simulink model "FirmwareArchitecture"  (R2024a)
settings: Solver=FixedStepDiscrete  StartTime=0.0  StopTime=10.0  RelTol=1e-3
model workspace (MAT data in the model file):
  AuralSystemInterface = Simulink.ServiceBus
  AuralSystemInterface.Elements_internal(1) = Simulink.FunctionElement
  AuralSystemInterface.Elements_internal(1).Prototype = 'vAuralSystemInit()'
  AuralSystemInterface.Elements_internal(1).Name = 'vAuralSystemInit'
  AuralSystemInterface.Elements_internal(1).Asynchronous = 0
  AuralSystemInterface.Elements_internal(2) = Simulink.FunctionElement
  AuralSystemInterface.Elements_internal(2).Prototype = 'vAuralSystemPlayWarningLevelChime()'
  AuralSystemInterface.Elements_internal(2).Name = 'vAuralSystemPlayWarningLevelChime'
  AuralSystemInterface.Elements_internal(2).Asynchronous = 0
  AuralSystemInterface.Elements_internal(3) = Simulink.FunctionElement
  AuralSystemInterface.Elements_internal(3).Prototype = 'vAuralSystemPlayFaultLevelChime()'
  AuralSystemInterface.Elements_internal(3).Name = 'vAuralSystemPlayFaultLevelChime'
  AuralSystemInterface.Elements_internal(3).Asynchronous = 0
  CollisionSensorInterface = Simulink.ServiceBus
  CollisionSensorInterface.Elements_internal(1) = Simulink.FunctionElement
  CollisionSensorInterface.Elements_internal(1).Prototype = 'vCollisionSensorInit(pCollisionCallBack)'
  CollisionSensorInterface.Elements_internal(1).Name = 'vCollisionSensorInit'
  CollisionSensorInterface.Elements_internal(1).Asynchronous = 0
  CollisionSensorInterface.Elements_internal(1).Arguments = Simulink.BusElement
  CollisionSensorInterface.Elements_internal(1).Arguments.DimensionsMode = 'Fixed'
  CollisionSensorInterface.Elements_internal(1).Arguments.SamplingMode = 'Sample based'
  CollisionSensorInterface.Elements_internal(1).Arguments.SampleTime = -1
  CollisionSensorInterface.Elements_internal(1).Arguments.Description = 'Pointer to Callback function'
  CollisionSensorInterface.Elements_internal(1).Arguments.Name = 'pCollisionCallBack'
  CollisionSensorInterface.Elements_internal(1).Arguments.DataType_internal = 'void (*)'
  CollisionSensorInterface.Elements_internal(1).Arguments.Complexity = 'real'
  CollisionSensorInterface.Elements_internal(1).Arguments.Dimensions = 1
  CollisionSensorInterface.Elements_internal(2) = Simulink.FunctionElement
  CollisionSensorInterface.Elements_internal(2).Prototype = 'vCollisionSensorDetectionHandler()'
  CollisionSensorInterface.Elements_internal(2).Name = 'vCollisionSensorDetectionHandler'
  CollisionSensorInterface.Elements_internal(2).Asynchronous = 0
  EncoderSystemInterface = Simulink.ServiceBus
  EncoderSystemInterface.Elements_internal(1) = Simulink.FunctionElement
  EncoderSystemInterface.Elements_internal(1).Prototype = 'vEncoderSystemInit(pLeftMotorCount,pRightMotorCount)'
  EncoderSystemInterface.Elements_internal(1).Name = 'vEncoderSystemInit'
  EncoderSystemInterface.Elements_internal(1).Asynchronous = 0
  EncoderSystemInterface.Elements_internal(1).Arguments(1) = Simulink.BusElement
  EncoderSystemInterface.Elements_internal(1).Arguments(1).DimensionsMode = 'Fixed'
  EncoderSystemInterface.Elements_internal(1).Arguments(1).SamplingMode = 'Sample based'
  EncoderSystemInterface.Elements_internal(1).Arguments(1).SampleTime = -1
  EncoderSystemInterface.Elements_internal(1).Arguments(1).Name = 'pLeftMotorCount'
  EncoderSystemInterface.Elements_internal(1).Arguments(1).DataType_internal = 'unsigned int*'
  EncoderSystemInterface.Elements_internal(1).Arguments(1).Complexity = 'real'
  EncoderSystemInterface.Elements_internal(1).Arguments(1).Dimensions = 1
  EncoderSystemInterface.Elements_internal(1).Arguments(2) = Simulink.BusElement
  EncoderSystemInterface.Elements_internal(1).Arguments(2).DimensionsMode = 'Fixed'
  EncoderSystemInterface.Elements_internal(1).Arguments(2).SamplingMode = 'Sample based'
  EncoderSystemInterface.Elements_internal(1).Arguments(2).SampleTime = -1
  EncoderSystemInterface.Elements_internal(1).Arguments(2).Name = 'pRightMotorCount'
  EncoderSystemInterface.Elements_internal(1).Arguments(2).DataType_internal = 'unsigned int*'
  EncoderSystemInterface.Elements_internal(1).Arguments(2).Complexity = 'real'
  EncoderSystemInterface.Elements_internal(1).Arguments(2).Dimensions = 1
  EncoderSystemInterface.Elements_internal(2) = Simulink.FunctionElement
  EncoderSystemInterface.Elements_internal(2).Prototype = 'vEncoderSystemExecuteMeasurement()'
  EncoderSystemInterface.Elements_internal(2).Name = 'vEncoderSystemExecuteMeasurement'
  EncoderSystemInterface.Elements_internal(2).Asynchronous = 0
  InfraredDistanceSystemInterface = Simulink.ServiceBus
  InfraredDistanceSystemInterface.Elements_internal(1) = Simulink.FunctionElement
  InfraredDistanceSystemInterface.Elements_internal(1).Prototype = 'vInfraredDistanceSystemInit(pDistanceMeasurement)'
  InfraredDistanceSystemInterface.Elements_internal(1).Name = 'vInfraredDistanceSystemInit'
  InfraredDistanceSystemInterface.Elements_internal(1).Asynchronous = 0
  InfraredDistanceSystemInterface.Elements_internal(1).Arguments = Simulink.BusElement
  InfraredDistanceSystemInterface.Elements_internal(1).Arguments.DimensionsMode = 'Fixed'
  InfraredDistanceSystemInterface.Elements_internal(1).Arguments.SamplingMode = 'Sample based'
  InfraredDistanceSystemInterface.Elements_internal(1).Arguments.SampleTime = -1
  InfraredDistanceSystemInterface.Elements_internal(1).Arguments.Name = 'pDistanceMeasurement'
  InfraredDistanceSystemInterface.Elements_internal(1).Arguments.DataType_internal = 'float*'
  InfraredDistanceSystemInterface.Elements_internal(1).Arguments.Complexity = 'real'
  InfraredDistanceSystemInterface.Elements_internal(1).Arguments.Dimensions = 1
  InfraredDistanceSystemInterface.Elements_internal(2) = Simulink.FunctionElement
  InfraredDistanceSystemInterface.Elements_internal(2).Prototype = 'vInfraredDistanceSystemExcecuteMeasurement()'
  InfraredDistanceSystemInterface.Elements_internal(2).Name = 'vInfraredDistanceSystemExcecuteMeasurement'
  InfraredDistanceSystemInterface.Elements_internal(2).Asynchronous = 0
  LineSensorSystemInterface = Simulink.ServiceBus
  LineSensorSystemInterface.Elements_internal = Simulink.FunctionElement
  LineSensorSystemInterface.Elements_internal.Prototype = 'LineSensorSystemInit(pLineSensorsReadings)'
  LineSensorSystemInterface.Elements_internal.Name = 'LineSensorSystemInit'
  LineSensorSystemInterface.Elements_internal.Asynchronous = 0
  LineSensorSystemInterface.Elements_internal.Arguments = Simulink.BusElement
  LineSensorSystemInterface.Elements_internal.Arguments.DimensionsMode = 'Fixed'
  LineSensorSystemInterface.Elements_internal.Arguments.SamplingMode = 'Sample based'
  LineSensorSystemInterface.Elements_internal.Arguments.SampleTime = -1
  LineSensorSystemInterface.Elements_internal.Arguments.Name = 'pLineSensorsReadings'
  LineSensorSystemInterface.Elements_internal.Arguments.DataType_internal = 'long unsigned int* [5]'
  LineSensorSystemInterface.Elements_internal.Arguments.Complexity = 'real'
  LineSensorSystemInterface.Elements_internal.Arguments.Dimensions = 5
  TelemetrySystemInterface = Simulink.ServiceBus
  TelemetrySystemInterface.Elements_internal(1) = Simulink.FunctionElement
  TelemetrySystemInterface.Elements_internal(1).Prototype = 'vTelemetrySystemInit()'
  TelemetrySystemInterface.Elements_internal(1).Name = 'vTelemetrySystemInit'
  TelemetrySystemInterface.Elements_internal(1).Asynchronous = 0
  TelemetrySystemInterface.Elements_internal(2) = Simulink.FunctionElement
  TelemetrySystemInterface.Elements_internal(2).Prototype = 'vTelemetrySystemSchedullingHandler(pTIM)'
  TelemetrySystemInterface.Elements_internal(2).Name = 'vTelemetrySystemSchedullingHandler'
  TelemetrySystemInterface.Elements_internal(2).Asynchronous = 1
  TelemetrySystemInterface.Elements_internal(2).Arguments = Simulink.BusElement
  TelemetrySystemInterface.Elements_internal(2).Arguments.DimensionsMode = 'Fixed'
  TelemetrySystemInterface.Elements_internal(2).Arguments.SamplingMode = 'Sample based'
  TelemetrySystemInterface.Elements_internal(2).Arguments.SampleTime = -1
  TelemetrySystemInterface.Elements_internal(2).Arguments.Name = 'pTIM'
  TelemetrySystemInterface.Elements_internal(2).Arguments.DataType_internal = 'TIM_HandleTypeDef*'
  TelemetrySystemInterface.Elements_internal(2).Arguments.Complexity = 'real'
  TelemetrySystemInterface.Elements_internal(2).Arguments.Dimensions = 1
  TelemetrySystemInterface.Elements_internal(3) = Simulink.FunctionElement
  TelemetrySystemInterface.Elements_internal(3).Prototype = 'vTelemetrySystemExternalEventHandler(uiGpioPin)'
  TelemetrySystemInterface.Elements_internal(3).Name = 'vTelemetrySystemExternalEventHandler'
  TelemetrySystemInterface.Elements_internal(3).Asynchronous = 1
  TelemetrySystemInterface.Elements_internal(3).Arguments = Simulink.BusElement
  TelemetrySystemInterface.Elements_internal(3).Arguments.DimensionsMode = 'Fixed'
  TelemetrySystemInterface.Elements_internal(3).Arguments.SamplingMode = 'Sample based'
  TelemetrySystemInterface.Elements_internal(3).Arguments.SampleTime = -1
  TelemetrySystemInterface.Elements_internal(3).Arguments.Name = 'uiGpioPin'
  TelemetrySystemInterface.Elements_internal(3).Arguments.DataType_internal = 'uint16'
  TelemetrySystemInterface.Elements_internal(3).Arguments.Complexity = 'real'
  TelemetrySystemInterface.Elements_internal(3).Arguments.Dimensions = 1
  UltrassonicDistanceSystemInterface = Simulink.ServiceBus
  UltrassonicDistanceSystemInterface.Elements_internal(1) = Simulink.FunctionElement
  UltrassonicDistanceSystemInterface.Elements_internal(1).Prototype = 'vUltrassonicDistanceSystemInit(pDistanceMeasurement)'
  UltrassonicDistanceSystemInterface.Elements_internal(1).Name = 'vUltrassonicDistanceSystemInit'
  UltrassonicDistanceSystemInterface.Elements_internal(1).Asynchronous = 0
  UltrassonicDistanceSystemInterface.Elements_internal(1).Arguments = Simulink.BusElement
  UltrassonicDistanceSystemInterface.Elements_internal(1).Arguments.DimensionsMode = 'Fixed'
  UltrassonicDistanceSystemInterface.Elements_internal(1).Arguments.SamplingMode = 'Sample based'
  UltrassonicDistanceSystemInterface.Elements_internal(1).Arguments.SampleTime = -1
  UltrassonicDistanceSystemInterface.Elements_internal(1).Arguments.Name = 'pDistanceMeasurement'
  UltrassonicDistanceSystemInterface.Elements_internal(1).Arguments.DataType_internal = 'float*'
  UltrassonicDistanceSystemInterface.Elements_internal(1).Arguments.Complexity = 'real'
  UltrassonicDistanceSystemInterface.Elements_internal(1).Arguments.Dimensions = 1
  UltrassonicDistanceSystemInterface.Elements_internal(2) = Simulink.FunctionElement
  UltrassonicDistanceSystemInterface.Elements_internal(2).Prototype = 'vUltrassonicDistanceSystemExecuteMeasurement()'
  UltrassonicDistanceSystemInterface.Elements_internal(2).Name = 'vUltrassonicDistanceSystemExecuteMeasurement'
  UltrassonicDistanceSystemInterface.Elements_internal(2).Asynchronous = 0
  UltrassonicDistanceSystemInterface.Elements_internal(3) = Simulink.FunctionElement
  UltrassonicDistanceSystemInterface.Elements_internal(3).Prototype = 'vUltrassonicDistanceSystemPulseHandler()'
  UltrassonicDistanceSystemInterface.Elements_internal(3).Name = 'vUltrassonicDistanceSystemPulseHandler'
  UltrassonicDistanceSystemInterface.Elements_internal(3).Asynchronous = 1
settings Model: Creator=pedro  LastModifiedBy=pedro

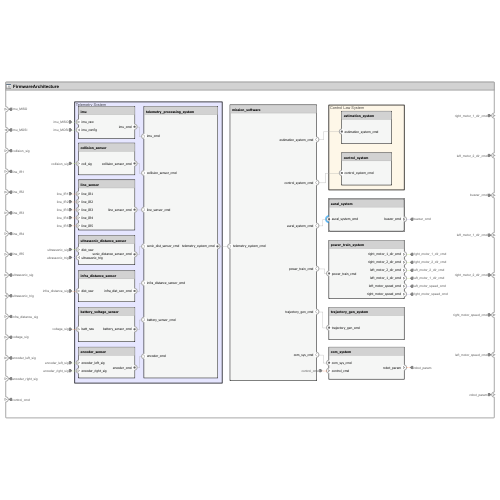
[thumbnail: Simulink's stored preview of the top-level diagram]
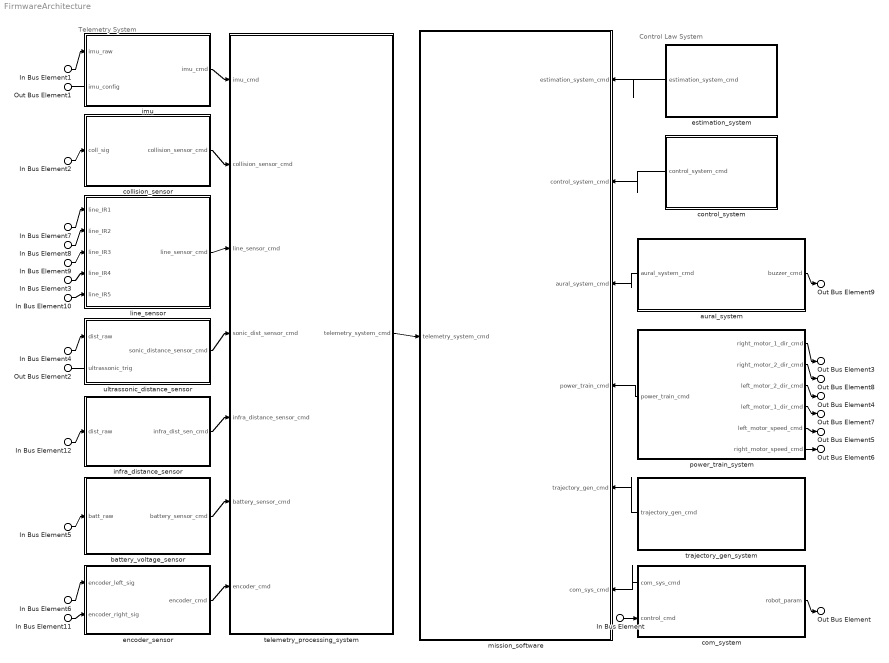
== system FirmwareArchitecture ==
  note: Control Law System
  note: Telemetry System
  In Bus Element1 : Inport  PortName=imu_MISO
  In Bus Element2 : Inport  Port=2  PortName=collision_sig
  In Bus Element7 : Inport  Port=3  PortName=line_IR1
  In Bus Element8 : Inport  Port=4  PortName=line_IR2
  In Bus Element9 : Inport  Port=5  PortName=line_IR3
  In Bus Element3 : Inport  Port=6  PortName=line_IR4
  In Bus Element10 : Inport  Port=7  PortName=line_IR5
  In Bus Element4 : Inport  Port=8  PortName=ultrassonic_sig
  In Bus Element5 : Inport  Port=9  PortName=voltage_sig
  In Bus Element12 : Inport  Port=10  PortName=infra_distance_sig
  In Bus Element6 : Inport  Port=11  PortName=encoder_left_sig
  In Bus Element11 : Inport  Port=12  PortName=encoder_right_sig
  In Bus Element : Inport  Port=13  PortName=control_cmd
  aural_system : Subsystem
      settings: PortSchema="{\"entries\":[{\"content\":{\"headerSize\":26,\"margin\":15,\"minimumSpacing\":25,\"sides\":[{\"content\":{\"connectorIds\":[\"Out2\"]},\"type\":\"ConnectorPlacement.EquallySpacedRectSide\",\"uuid\":\"4d6c5e10-6186-41fb-b2bf-ba98d7aba04e\"},{\"content\":{\"connectorIds\":[\"Out1\"],\"side\":\"RIGHT\"},\"type\":\"ConnectorPlacement.EquallySpacedRectSide\",\"uuid\":\"376cbcb5-ae00-4ee4-b51a-d7e41488d4d0\"},{\"content\":{\"side\":\"TOP\"},\"type\":\"ConnectorPlacement.EquallySpacedRectSide\",\"uuid\":\"7d78b6f2-ded8-4819-b676-701e54dd8720\"}]},\"type\":\"ConnectorPlacement.EquallySpacedConnector\",\"uuid\":\"61036d85-7ed2-4698-95df-f6a26735d595\"}],\"packageUris\":[\"http://schema.mathworks.com/mf0/Connector/R2020b\"],\"version\":\"1.0\"}"
  battery_voltage_sensor : Subsystem
      settings: PortSchema="{\"entries\":[{\"content\":{\"headerSize\":26,\"margin\":15,\"minimumSpacing\":25,\"sides\":[{\"content\":{\"connectorIds\":[\"In1\"]},\"type\":\"ConnectorPlacement.EquallySpacedRectSide\",\"uuid\":\"4d6c5e10-6186-41fb-b2bf-ba98d7aba04e\"},{\"content\":{\"connectorIds\":[\"Out1\"],\"side\":\"RIGHT\"},\"type\":\"ConnectorPlacement.EquallySpacedRectSide\",\"uuid\":\"376cbcb5-ae00-4ee4-b51a-d7e41488d4d0\"},{\"content\":{\"side\":\"TOP\"},\"type\":\"ConnectorPlacement.EquallySpacedRectSide\",\"uuid\":\"7d78b6f2-ded8-4819-b676-701e54dd8720\"}]},\"type\":\"ConnectorPlacement.EquallySpacedConnector\",\"uuid\":\"61036d85-7ed2-4698-95df-f6a26735d595\"}],\"packageUris\":[\"http://schema.mathworks.com/mf0/Connector/R2020b\"],\"version\":\"1.0\"}"
  collision_sensor : Subsystem
      settings: PortSchema="{\"entries\":[{\"content\":{\"headerSize\":26,\"margin\":15,\"minimumSpacing\":25,\"sides\":[{\"content\":{\"connectorIds\":[\"In1\"]},\"type\":\"ConnectorPlacement.EquallySpacedRectSide\",\"uuid\":\"4d6c5e10-6186-41fb-b2bf-ba98d7aba04e\"},{\"content\":{\"connectorIds\":[\"Out1\"],\"side\":\"RIGHT\"},\"type\":\"ConnectorPlacement.EquallySpacedRectSide\",\"uuid\":\"376cbcb5-ae00-4ee4-b51a-d7e41488d4d0\"},{\"content\":{\"side\":\"TOP\"},\"type\":\"ConnectorPlacement.EquallySpacedRectSide\",\"uuid\":\"7d78b6f2-ded8-4819-b676-701e54dd8720\"}]},\"type\":\"ConnectorPlacement.EquallySpacedConnector\",\"uuid\":\"61036d85-7ed2-4698-95df-f6a26735d595\"}],\"packageUris\":[\"http://schema.mathworks.com/mf0/Connector/R2020b\"],\"version\":\"1.0\"}"
  com_system : Subsystem
      settings: PortSchema="{\"entries\":[{\"content\":{\"headerSize\":26,\"margin\":15,\"minimumSpacing\":25,\"sides\":[{\"content\":{\"connectorIds\":[\"Out2\",\"In1\"]},\"type\":\"ConnectorPlacement.EquallySpacedRectSide\",\"uuid\":\"4d6c5e10-6186-41fb-b2bf-ba98d7aba04e\"},{\"content\":{\"connectorIds\":[\"Out1\"],\"side\":\"RIGHT\"},\"type\":\"ConnectorPlacement.EquallySpacedRectSide\",\"uuid\":\"376cbcb5-ae00-4ee4-b51a-d7e41488d4d0\"},{\"content\":{\"side\":\"TOP\"},\"type\":\"ConnectorPlacement.EquallySpacedRectSide\",\"uuid\":\"7d78b6f2-ded8-4819-b676-701e54dd8720\"}]},\"type\":\"ConnectorPlacement.EquallySpacedConnector\",\"uuid\":\"61036d85-7ed2-4698-95df-f6a26735d595\"}],\"packageUris\":[\"http://schema.mathworks.com/mf0/Connector/R2020b\"],\"version\":\"1.0\"}"
  control_system : Subsystem
      settings: PortSchema="{\"entries\":[{\"content\":{\"headerSize\":26,\"margin\":15,\"minimumSpacing\":25,\"sides\":[{\"content\":{\"connectorIds\":[\"Out1\"]},\"type\":\"ConnectorPlacement.EquallySpacedRectSide\",\"uuid\":\"4d6c5e10-6186-41fb-b2bf-ba98d7aba04e\"},{\"content\":{\"side\":\"RIGHT\"},\"type\":\"ConnectorPlacement.EquallySpacedRectSide\",\"uuid\":\"376cbcb5-ae00-4ee4-b51a-d7e41488d4d0\"},{\"content\":{\"side\":\"TOP\"},\"type\":\"ConnectorPlacement.EquallySpacedRectSide\",\"uuid\":\"7d78b6f2-ded8-4819-b676-701e54dd8720\"}]},\"type\":\"ConnectorPlacement.EquallySpacedConnector\",\"uuid\":\"61036d85-7ed2-4698-95df-f6a26735d595\"}],\"packageUris\":[\"http://schema.mathworks.com/mf0/Connector/R2020b\"],\"version\":\"1.0\"}"
  encoder_sensor : Subsystem
      settings: PortSchema="{\"entries\":[{\"content\":{\"headerSize\":26,\"margin\":15,\"minimumSpacing\":25,\"sides\":[{\"content\":{\"connectorIds\":[\"In1\",\"In2\"]},\"type\":\"ConnectorPlacement.EquallySpacedRectSide\",\"uuid\":\"4d6c5e10-6186-41fb-b2bf-ba98d7aba04e\"},{\"content\":{\"connectorIds\":[\"Out1\"],\"side\":\"RIGHT\"},\"type\":\"ConnectorPlacement.EquallySpacedRectSide\",\"uuid\":\"376cbcb5-ae00-4ee4-b51a-d7e41488d4d0\"},{\"content\":{\"side\":\"TOP\"},\"type\":\"ConnectorPlacement.EquallySpacedRectSide\",\"uuid\":\"7d78b6f2-ded8-4819-b676-701e54dd8720\"}]},\"type\":\"ConnectorPlacement.EquallySpacedConnector\",\"uuid\":\"61036d85-7ed2-4698-95df-f6a26735d595\"}],\"packageUris\":[\"http://schema.mathworks.com/mf0/Connector/R2020b\"],\"version\":\"1.0\"}"
  estimation_system : Subsystem
      settings: PortSchema="{\"entries\":[{\"content\":{\"headerSize\":26,\"margin\":15,\"minimumSpacing\":25,\"sides\":[{\"content\":{\"connectorIds\":[\"Out1\"]},\"type\":\"ConnectorPlacement.EquallySpacedRectSide\",\"uuid\":\"4d6c5e10-6186-41fb-b2bf-ba98d7aba04e\"},{\"content\":{\"side\":\"RIGHT\"},\"type\":\"ConnectorPlacement.EquallySpacedRectSide\",\"uuid\":\"376cbcb5-ae00-4ee4-b51a-d7e41488d4d0\"},{\"content\":{\"side\":\"TOP\"},\"type\":\"ConnectorPlacement.EquallySpacedRectSide\",\"uuid\":\"7d78b6f2-ded8-4819-b676-701e54dd8720\"}]},\"type\":\"ConnectorPlacement.EquallySpacedConnector\",\"uuid\":\"61036d85-7ed2-4698-95df-f6a26735d595\"}],\"packageUris\":[\"http://schema.mathworks.com/mf0/Connector/R2020b\"],\"version\":\"1.0\"}"
  imu : Subsystem
      settings: PortSchema="{\"entries\":[{\"content\":{\"headerSize\":26,\"margin\":15,\"minimumSpacing\":25,\"sides\":[{\"content\":{\"connectorIds\":[\"In1\",\"Out2\"]},\"type\":\"ConnectorPlacement.EquallySpacedRectSide\",\"uuid\":\"4d6c5e10-6186-41fb-b2bf-ba98d7aba04e\"},{\"content\":{\"connectorIds\":[\"Out1\"],\"side\":\"RIGHT\"},\"type\":\"ConnectorPlacement.EquallySpacedRectSide\",\"uuid\":\"376cbcb5-ae00-4ee4-b51a-d7e41488d4d0\"},{\"content\":{\"side\":\"TOP\"},\"type\":\"ConnectorPlacement.EquallySpacedRectSide\",\"uuid\":\"7d78b6f2-ded8-4819-b676-701e54dd8720\"}]},\"type\":\"ConnectorPlacement.EquallySpacedConnector\",\"uuid\":\"61036d85-7ed2-4698-95df-f6a26735d595\"}],\"packageUris\":[\"http://schema.mathworks.com/mf0/Connector/R2020b\"],\"version\":\"1.0\"}"
  infra_distance_sensor : Subsystem
      settings: PortSchema="{\"entries\":[{\"content\":{\"headerSize\":26,\"margin\":15,\"minimumSpacing\":25,\"sides\":[{\"content\":{\"connectorIds\":[\"In1\"]},\"type\":\"ConnectorPlacement.EquallySpacedRectSide\",\"uuid\":\"4d6c5e10-6186-41fb-b2bf-ba98d7aba04e\"},{\"content\":{\"connectorIds\":[\"Out1\"],\"side\":\"RIGHT\"},\"type\":\"ConnectorPlacement.EquallySpacedRectSide\",\"uuid\":\"376cbcb5-ae00-4ee4-b51a-d7e41488d4d0\"},{\"content\":{\"side\":\"TOP\"},\"type\":\"ConnectorPlacement.EquallySpacedRectSide\",\"uuid\":\"7d78b6f2-ded8-4819-b676-701e54dd8720\"}]},\"type\":\"ConnectorPlacement.EquallySpacedConnector\",\"uuid\":\"61036d85-7ed2-4698-95df-f6a26735d595\"}],\"packageUris\":[\"http://schema.mathworks.com/mf0/Connector/R2020b\"],\"version\":\"1.0\"}"
  line_sensor : Subsystem
      settings: PortSchema="{\"entries\":[{\"content\":{\"headerSize\":26,\"margin\":15,\"minimumSpacing\":25,\"sides\":[{\"content\":{\"connectorIds\":[\"In1\",\"In2\",\"In3\",\"In4\",\"In5\"]},\"type\":\"ConnectorPlacement.EquallySpacedRectSide\",\"uuid\":\"4d6c5e10-6186-41fb-b2bf-ba98d7aba04e\"},{\"content\":{\"connectorIds\":[\"Out1\"],\"side\":\"RIGHT\"},\"type\":\"ConnectorPlacement.EquallySpacedRectSide\",\"uuid\":\"376cbcb5-ae00-4ee4-b51a-d7e41488d4d0\"},{\"content\":{\"side\":\"TOP\"},\"type\":\"ConnectorPlacement.EquallySpacedRectSide\",\"uuid\":\"7d78b6f2-ded8-4819-b676-701e54dd8720\"}]},\"type\":\"ConnectorPlacement.EquallySpacedConnector\",\"uuid\":\"61036d85-7ed2-4698-95df-f6a26735d595\"}],\"packageUris\":[\"http://schema.mathworks.com/mf0/Connector/R2020b\"],\"version\":\"1.0\"}"
  mission_software : Subsystem
      settings: PortSchema="{\"entries\":[{\"content\":{\"headerSize\":26,\"margin\":15,\"minimumSpacing\":25,\"sides\":[{\"content\":{\"connectorIds\":[\"In6\"]},\"type\":\"ConnectorPlacement.EquallySpacedRectSide\",\"uuid\":\"4d6c5e10-6186-41fb-b2bf-ba98d7aba04e\"},{\"content\":{\"connectorIds\":[\"In1\",\"In2\",\"In3\",\"In4\",\"In5\",\"In7\"],\"side\":\"RIGHT\"},\"type\":\"ConnectorPlacement.EquallySpacedRectSide\",\"uuid\":\"376cbcb5-ae00-4ee4-b51a-d7e41488d4d0\"},{\"content\":{\"side\":\"TOP\"},\"type\":\"ConnectorPlacement.EquallySpacedRectSide\",\"uuid\":\"7d78b6f2-ded8-4819-b676-701e54dd8720\"}]},\"type\":\"ConnectorPlacement.EquallySpacedConnector\",\"uuid\":\"61036d85-7ed2-4698-95df-f6a26735d595\"}],\"packageUris\":[\"http://schema.mathworks.com/mf0/Connector/R2020b\"],\"version\":\"1.0\"}"
  power_train_system : Subsystem
      settings: PortSchema="{\"entries\":[{\"content\":{\"headerSize\":26,\"margin\":15,\"minimumSpacing\":25,\"sides\":[{\"content\":{\"connectorIds\":[\"Out7\"]},\"type\":\"ConnectorPlacement.EquallySpacedRectSide\",\"uuid\":\"4d6c5e10-6186-41fb-b2bf-ba98d7aba04e\"},{\"content\":{\"connectorIds\":[\"Out1\",\"Out4\",\"Out2\",\"Out3\",\"Out6\",\"Out5\"],\"side\":\"RIGHT\"},\"type\":\"ConnectorPlacement.EquallySpacedRectSide\",\"uuid\":\"376cbcb5-ae00-4ee4-b51a-d7e41488d4d0\"},{\"content\":{\"side\":\"TOP\"},\"type\":\"ConnectorPlacement.EquallySpacedRectSide\",\"uuid\":\"7d78b6f2-ded8-4819-b676-701e54dd8720\"}]},\"type\":\"ConnectorPlacement.EquallySpacedConnector\",\"uuid\":\"61036d85-7ed2-4698-95df-f6a26735d595\"}],\"packageUris\":[\"http://schema.mathworks.com/mf0/Connector/R2020b\"],\"version\":\"1.0\"}"
  telemetry_processing_system : Subsystem
      settings: PortSchema="{\"entries\":[{\"content\":{\"headerSize\":26,\"margin\":15,\"minimumSpacing\":25,\"sides\":[{\"content\":{\"connectorIds\":[\"In1\",\"In3\",\"In2\",\"In4\",\"In5\",\"In6\",\"In7\"]},\"type\":\"ConnectorPlacement.EquallySpacedRectSide\",\"uuid\":\"4d6c5e10-6186-41fb-b2bf-ba98d7aba04e\"},{\"content\":{\"connectorIds\":[\"Out1\"],\"side\":\"RIGHT\"},\"type\":\"ConnectorPlacement.EquallySpacedRectSide\",\"uuid\":\"376cbcb5-ae00-4ee4-b51a-d7e41488d4d0\"},{\"content\":{\"side\":\"TOP\"},\"type\":\"ConnectorPlacement.EquallySpacedRectSide\",\"uuid\":\"7d78b6f2-ded8-4819-b676-701e54dd8720\"}]},\"type\":\"ConnectorPlacement.EquallySpacedConnector\",\"uuid\":\"61036d85-7ed2-4698-95df-f6a26735d595\"}],\"packageUris\":[\"http://schema.mathworks.com/mf0/Connector/R2020b\"],\"version\":\"1.0\"}"
  trajectory_gen_system : Subsystem
      settings: PortSchema="{\"entries\":[{\"content\":{\"headerSize\":26,\"margin\":15,\"minimumSpacing\":25,\"sides\":[{\"content\":{\"connectorIds\":[\"Out1\"]},\"type\":\"ConnectorPlacement.EquallySpacedRectSide\",\"uuid\":\"4d6c5e10-6186-41fb-b2bf-ba98d7aba04e\"},{\"content\":{\"side\":\"RIGHT\"},\"type\":\"ConnectorPlacement.EquallySpacedRectSide\",\"uuid\":\"376cbcb5-ae00-4ee4-b51a-d7e41488d4d0\"},{\"content\":{\"side\":\"TOP\"},\"type\":\"ConnectorPlacement.EquallySpacedRectSide\",\"uuid\":\"7d78b6f2-ded8-4819-b676-701e54dd8720\"}]},\"type\":\"ConnectorPlacement.EquallySpacedConnector\",\"uuid\":\"61036d85-7ed2-4698-95df-f6a26735d595\"}],\"packageUris\":[\"http://schema.mathworks.com/mf0/Connector/R2020b\"],\"version\":\"1.0\"}"
  ultrassonic_distance_sensor : Subsystem
      settings: PortSchema="{\"entries\":[{\"content\":{\"headerSize\":26,\"margin\":15,\"minimumSpacing\":25,\"sides\":[{\"content\":{\"connectorIds\":[\"In1\",\"Out2\"]},\"type\":\"ConnectorPlacement.EquallySpacedRectSide\",\"uuid\":\"4d6c5e10-6186-41fb-b2bf-ba98d7aba04e\"},{\"content\":{\"connectorIds\":[\"Out1\"],\"side\":\"RIGHT\"},\"type\":\"ConnectorPlacement.EquallySpacedRectSide\",\"uuid\":\"376cbcb5-ae00-4ee4-b51a-d7e41488d4d0\"},{\"content\":{\"side\":\"TOP\"},\"type\":\"ConnectorPlacement.EquallySpacedRectSide\",\"uuid\":\"7d78b6f2-ded8-4819-b676-701e54dd8720\"}]},\"type\":\"ConnectorPlacement.EquallySpacedConnector\",\"uuid\":\"61036d85-7ed2-4698-95df-f6a26735d595\"}],\"packageUris\":[\"http://schema.mathworks.com/mf0/Connector/R2020b\"],\"version\":\"1.0\"}"
  Out Bus Element1 : Outport  PortName=imu_MOSI
  Out Bus Element3 : Outport  Port=2  PortName=right_motor_1_dir_cmd
  Out Bus Element4 : Outport  Port=3  PortName=left_motor_2_dir_cmd
  Out Bus Element9 : Outport  Port=4  PortName=buzzer_cmd
  Out Bus Element7 : Outport  Port=5  PortName=left_motor_1_dir_cmd
  Out Bus Element8 : Outport  Port=6  PortName=right_motor_2_dir_cmd
  Out Bus Element6 : Outport  Port=7  PortName=right_motor_speed_cmd
  Out Bus Element5 : Outport  Port=8  PortName=left_motor_speed_cmd
  Out Bus Element2 : Outport  Port=9  PortName=ultrassonic_trig
  Out Bus Element : Outport  Port=10  PortName=robot_param
  wires:
  imu/1(imu_cmd) -> telemetry_processing_system/1(imu_cmd)
  collision_sensor/1(collision_sensor_cmd) -> telemetry_processing_system/3(collision_sensor_cmd)
  line_sensor/1(line_sensor_cmd) -> telemetry_processing_system/2(line_sensor_cmd)
  ultrassonic_distance_sensor/1(sonic_distance_sensor_cmd) -> telemetry_processing_system/4(sonic_dist_sensor_cmd)
  battery_voltage_sensor/1(battery_sensor_cmd) -> telemetry_processing_system/6(battery_sensor_cmd)
  encoder_sensor/1(encoder_cmd) -> telemetry_processing_system/7(encoder_cmd)
  com_system/2(com_sys_cmd) -> mission_software/7(com_sys_cmd)
  telemetry_processing_system/1(telemetry_system_cmd) -> mission_software/6(telemetry_system_cmd)
  estimation_system/1(estimation_system_cmd) -> mission_software/1(estimation_system_cmd)
  control_system/1(control_system_cmd) -> mission_software/2(control_system_cmd)
  trajectory_gen_system/1(trajectory_gen_cmd) -> mission_software/5(trajectory_gen_cmd)
  com_system/1(robot_param) -> Out Bus Element/1
  In Bus Element/1 -> com_system/1(control_cmd)
  In Bus Element1/1 -> imu/1(imu_raw)
  In Bus Element2/1 -> collision_sensor/1(coll_sig)
  In Bus Element3/1 -> line_sensor/4(line_IR4)
  In Bus Element4/1 -> ultrassonic_distance_sensor/1(dist_raw)
  In Bus Element5/1 -> battery_voltage_sensor/1(batt_raw)
  In Bus Element6/1 -> encoder_sensor/1(encoder_left_sig)
  imu/2(imu_config) -> Out Bus Element1/1
  In Bus Element7/1 -> line_sensor/1(line_IR1)
  In Bus Element8/1 -> line_sensor/2(line_IR2)
  In Bus Element9/1 -> line_sensor/3(line_IR3)
  In Bus Element10/1 -> line_sensor/5(line_IR5)
  ultrassonic_distance_sensor/2(ultrassonic_trig) -> Out Bus Element2/1
  In Bus Element11/1 -> encoder_sensor/2(encoder_right_sig)
  power_train_system/1(right_motor_1_dir_cmd) -> Out Bus Element3/1
  power_train_system/2(left_motor_2_dir_cmd) -> Out Bus Element4/1
  power_train_system/6(left_motor_speed_cmd) -> Out Bus Element5/1
  power_train_system/5(right_motor_speed_cmd) -> Out Bus Element6/1
  power_train_system/7(power_train_cmd) -> mission_software/4(power_train_cmd)
  infra_distance_sensor/1(infra_dist_sen_cmd) -> telemetry_processing_system/5(infra_distance_sensor_cmd)
  In Bus Element12/1 -> infra_distance_sensor/1(dist_raw)
  power_train_system/3(left_motor_1_dir_cmd) -> Out Bus Element7/1
  power_train_system/4(right_motor_2_dir_cmd) -> Out Bus Element8/1
  aural_system/2(aural_system_cmd) -> mission_software/3(aural_system_cmd)
  aural_system/1(buzzer_cmd) -> Out Bus Element9/1

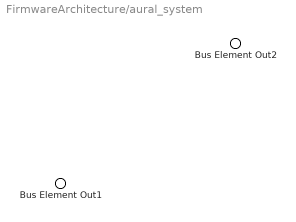
== system FirmwareArchitecture/aural_system ==
  Bus Element Out2 : Outport  PortName=buzzer_cmd
  Bus Element Out1 : Outport  Port=2  AllowServiceAccess=on  PortName=aural_system_cmd

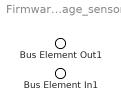
== system FirmwareArchitecture/battery_voltage_sensor ==
  Bus Element In1 : Inport  PortName=batt_raw
  Bus Element Out1 : Outport  AllowServiceAccess=on  PortName=battery_sensor_cmd

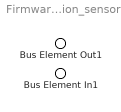
== system FirmwareArchitecture/collision_sensor ==
  Bus Element In1 : Inport  PortName=coll_sig
  Bus Element Out1 : Outport  AllowServiceAccess=on  PortName=collision_sensor_cmd

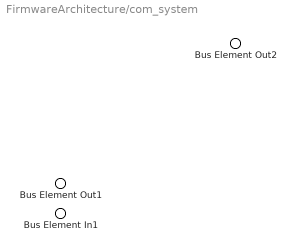
== system FirmwareArchitecture/com_system ==
  Bus Element In1 : Inport  PortName=control_cmd
  Bus Element Out2 : Outport  PortName=robot_param
  Bus Element Out1 : Outport  Port=2  AllowServiceAccess=on  PortName=com_sys_cmd

== system FirmwareArchitecture/control_system ==
  Bus Element Out1 : Outport  AllowServiceAccess=on  PortName=control_system_cmd

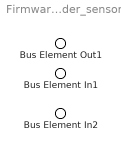
== system FirmwareArchitecture/encoder_sensor ==
  Bus Element In1 : Inport  PortName=encoder_left_sig
  Bus Element In2 : Inport  Port=2  PortName=encoder_right_sig
  Bus Element Out1 : Outport  AllowServiceAccess=on  PortName=encoder_cmd

== system FirmwareArchitecture/estimation_system ==
  Bus Element Out1 : Outport  AllowServiceAccess=on  PortName=estimation_system_cmd

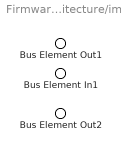
== system FirmwareArchitecture/imu ==
  Bus Element In1 : Inport  PortName=imu_raw
  Bus Element Out1 : Outport  AllowServiceAccess=on  PortName=imu_cmd
  Bus Element Out2 : Outport  Port=2  PortName=imu_config

== system FirmwareArchitecture/infra_distance_sensor ==
  Bus Element In1 : Inport  PortName=dist_raw
  Bus Element Out1 : Outport  AllowServiceAccess=on  PortName=infra_dist_sen_cmd

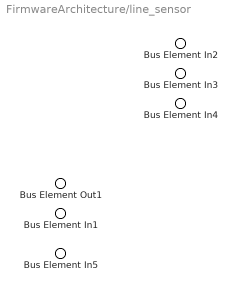
== system FirmwareArchitecture/line_sensor ==
  Bus Element In2 : Inport  PortName=line_IR1
  Bus Element In3 : Inport  Port=2  PortName=line_IR2
  Bus Element In4 : Inport  Port=3  PortName=line_IR3
  Bus Element In1 : Inport  Port=4  PortName=line_IR4
  Bus Element In5 : Inport  Port=5  PortName=line_IR5
  Bus Element Out1 : Outport  AllowServiceAccess=on  PortName=line_sensor_cmd

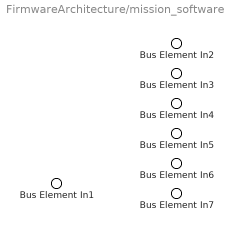
== system FirmwareArchitecture/mission_software ==
  Bus Element In3 : Inport  AllowServiceAccess=on  PortName=estimation_system_cmd
  Bus Element In4 : Inport  Port=2  AllowServiceAccess=on  PortName=control_system_cmd
  Bus Element In7 : Inport  Port=3  AllowServiceAccess=on  PortName=aural_system_cmd
  Bus Element In6 : Inport  Port=4  AllowServiceAccess=on  PortName=power_train_cmd
  Bus Element In5 : Inport  Port=5  AllowServiceAccess=on  PortName=trajectory_gen_cmd
  Bus Element In2 : Inport  Port=6  AllowServiceAccess=on  PortName=telemetry_system_cmd
  Bus Element In1 : Inport  Port=7  AllowServiceAccess=on  PortName=com_sys_cmd

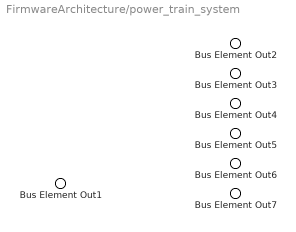
== system FirmwareArchitecture/power_train_system ==
  Bus Element Out2 : Outport  PortName=right_motor_1_dir_cmd
  Bus Element Out3 : Outport  Port=2  PortName=left_motor_2_dir_cmd
  Bus Element Out6 : Outport  Port=3  PortName=left_motor_1_dir_cmd
  Bus Element Out7 : Outport  Port=4  PortName=right_motor_2_dir_cmd
  Bus Element Out5 : Outport  Port=5  PortName=right_motor_speed_cmd
  Bus Element Out4 : Outport  Port=6  PortName=left_motor_speed_cmd
  Bus Element Out1 : Outport  Port=7  AllowServiceAccess=on  PortName=power_train_cmd

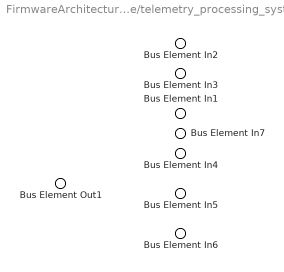
== system FirmwareArchitecture/telemetry_processing_system ==
  Bus Element In2 : Inport  AllowServiceAccess=on  PortName=imu_cmd
  Bus Element In3 : Inport  Port=2  AllowServiceAccess=on  PortName=line_sensor_cmd
  Bus Element In1 : Inport  Port=3  AllowServiceAccess=on  PortName=collision_sensor_cmd
  Bus Element In4 : Inport  Port=4  AllowServiceAccess=on  PortName=sonic_dist_sensor_cmd
  Bus Element In7 : Inport  Port=5  AllowServiceAccess=on  PortName=infra_distance_sensor_cmd
  Bus Element In5 : Inport  Port=6  AllowServiceAccess=on  PortName=battery_sensor_cmd
  Bus Element In6 : Inport  Port=7  AllowServiceAccess=on  PortName=encoder_cmd
  Bus Element Out1 : Outport  AllowServiceAccess=on  PortName=telemetry_system_cmd

== system FirmwareArchitecture/trajectory_gen_system ==
  Bus Element Out1 : Outport  AllowServiceAccess=on  PortName=trajectory_gen_cmd

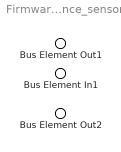
== system FirmwareArchitecture/ultrassonic_distance_sensor ==
  Bus Element In1 : Inport  PortName=dist_raw
  Bus Element Out1 : Outport  AllowServiceAccess=on  PortName=sonic_distance_sensor_cmd
  Bus Element Out2 : Outport  Port=2  PortName=ultrassonic_trig
